simulink model "fsm_12B_with_contracts"  (R2019b)
settings: Solver=FixedStepDiscrete  StartTime=0.0  StopTime=10  RelTol=1e-3  EnableMultiTasking=on
model workspace (MAT data in the model file):
  ContractValidatorBlocksMap : containers.Map (value not decoded)
undefined symbols (not defined in the file): contractAfterSimulation, contractBeforeSimulation, ContractBlock, ContractGuaranteeBlock, ContractValidatorBlock, saveValidatorParameters
libraries: cocosimLibs x20
(part 1 of 2)
settings Model: Creator=elliocm  LastModifiedBy=hbourbou
settings DataIOCC: LimitDataPoints=on  SaveFormat=Array  ReturnWorkspaceOutputs=off
settings OptimizationCC: ExpressionDepthLimit=2147483647  LifeSpan=inf
settings DebuggingCC: UnderspecifiedInitializationDetection=Classic  MergeDetectMultiDrivingBlocksExec=none  SolverPrmCheckMsg=warning  StateNameClashWarn=warning  SFUnexpectedBacktrackingDiag=warning  SFNoUnconditionalDefaultTransitionDiag=warning  SFExecutionAtInitializationDiag=none  ArithmeticOperatorsInVariantConditions=warning
settings HardwareCC: ProdBitPerPointer=32  ProdBitPerSizeT=32  ProdBitPerPtrDiffT=32  ProdLargestAtomicFloat=None  ProdIntDivRoundTo=Undefined  ProdEndianess=Unspecified  ProdWordSize=32  ProdHWDeviceType=32-bit Generic
settings ModelReferenceCC: PropagateSignalLabelsOutOfModel=off
settings SFSimCC: SimUseLocalCustomCode=off  CustomCodeUndefinedFunction=UseInterfaceOnly
settings RTWCC: RTWUseLocalCustomCode=off
settings CodeAppCC: StateflowObjectComments=on
settings GRTTargetCC: TargetLangStandard=C89/C90 (ANSI)  GeneratePreprocessorConditionals=Disable all
settings ConfigComp: CovMetricSettings=dw  CovHtmlReporting=on  CovSaveCumulativeToWorkspaceVar=on  CovSaveSingleToWorkspaceVar=on  CovExternalEMLEnable=off

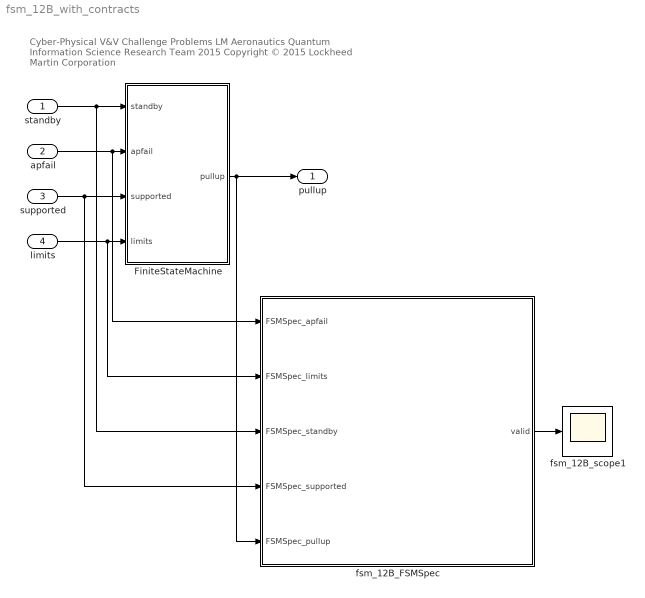
== system fsm_12B_with_contracts ==
  note: Cyber-Physical V&V Challenge Problems
      | LM Aeronautics Quantum Information Science Research Team 2015
      | Copyright © 2015 Lockheed Martin Corporation
  standby : Inport  OutDataTypeStr=boolean
  apfail : Inport  Port=2  OutDataTypeStr=boolean
  supported : Inport  Port=3  OutDataTypeStr=boolean
  limits : Inport  Port=4  OutDataTypeStr=boolean
  FiniteStateMachine : Subsystem
  fsm_12B_FSMSpec : Subsystem  mask(ContractBlock){ContractBlockType=ContractBlock}
      mask init:
      | set_param(gcb, 'LinkStatus', 'none');
      mask DialogControl DescTextVar Prompt: Contract block
      mask Display:
      | text(0.5, 0.5, '{\bf\fontsize{20}Contract}', 'hor', 'center', 'texmode','on');
      | blocks = find_system(gcb, 'LookUnderMasks','all', 'SearchDepth',1,'BlockType','Inport');
      | for i = 1 : length(blocks)
      |     blockName = get_param(blocks(i), 'Name');
      |     [path, blockName] = fileparts(char(blockName));
      |     port_label('input', i, blockName);
      | end
      | 
      | blocks = find_system(gcb, 'LookUnderMasks','all', 'SearchDepth',1,'BlockType','Outport');
      | for i = 1 : length(blocks)
      |     blockName = get_param(blocks(i), 'Name');
      |     [path, blockName] = fileparts(char(blockName));
      |     port_label('output', i, blockName);
      | end
  fsm_12B_scope1 : Scope
  pullup : Outport  VectorParamsAs1DForOutWhenUnconnected=off
  wires:
  standby/1 -> FiniteStateMachine/1(standby), fsm_12B_FSMSpec/3(FSMSpec_standby)
  apfail/1 -> FiniteStateMachine/2(apfail), fsm_12B_FSMSpec/1(FSMSpec_apfail)
  supported/1 -> FiniteStateMachine/3(supported), fsm_12B_FSMSpec/4(FSMSpec_supported)
  limits/1 -> FiniteStateMachine/4(limits), fsm_12B_FSMSpec/2(FSMSpec_limits)
  FiniteStateMachine/1(pullup) -> pullup/1, fsm_12B_FSMSpec/5(FSMSpec_pullup)
  fsm_12B_FSMSpec/1(valid) -> fsm_12B_scope1/1

== system fsm_12B_with_contracts/FiniteStateMachine ==
  note: 51
  standby : Inport
  apfail : Inport  Port=2
  supported : Inport  Port=3
  limits : Inport  Port=4
  FiniteStateMachine_FSM_AutopilotSpec1 : Subsystem  mask(ContractBlock){ContractBlockType=ContractBlock}
      mask init:
      | set_param(gcb, 'LinkStatus', 'none');
      mask DialogControl DescTextVar Prompt: Contract block
      mask Display:
      | text(0.5, 0.5, '{\bf\fontsize{20}Contract}', 'hor', 'center', 'texmode','on');
      | blocks = find_system(gcb, 'LookUnderMasks','all', 'SearchDepth',1,'BlockType','Inport');
      | for i = 1 : length(blocks)
      |     blockName = get_param(blocks(i), 'Name');
      |     [path, blockName] = fileparts(char(blockName));
      |     port_label('input', i, blockName);
      | end
      | 
      | blocks = find_system(gcb, 'LookUnderMasks','all', 'SearchDepth',1,'BlockType','Outport');
      | for i = 1 : length(blocks)
      |     blockName = get_param(blocks(i), 'Name');
      |     [path, blockName] = fileparts(char(blockName));
      |     port_label('output', i, blockName);
      | end
  FiniteStateMachine_FSM_SensorSpec : Subsystem  mask(ContractBlock){ContractBlockType=ContractBlock}
      mask init:
      | set_param(gcb, 'LinkStatus', 'none');
      mask DialogControl DescTextVar Prompt: Contract block
      mask Display:
      | text(0.5, 0.5, '{\bf\fontsize{20}Contract}', 'hor', 'center', 'texmode','on');
      | blocks = find_system(gcb, 'LookUnderMasks','all', 'SearchDepth',1,'BlockType','Inport');
      | for i = 1 : length(blocks)
      |     blockName = get_param(blocks(i), 'Name');
      |     [path, blockName] = fileparts(char(blockName));
      |     port_label('input', i, blockName);
      | end
      | 
      | blocks = find_system(gcb, 'LookUnderMasks','all', 'SearchDepth',1,'BlockType','Outport');
      | for i = 1 : length(blocks)
      |     blockName = get_param(blocks(i), 'Name');
      |     [path, blockName] = fileparts(char(blockName));
      |     port_label('output', i, blockName);
      | end
  Manager : Subsystem
  Sen : Subsystem
  Terminator : Terminator
  Terminator1 : Terminator
  Unit Delay : UnitDelay  SampleTime=-1  HasFrameUpgradeWarning=on
  Unit Delay1 : UnitDelay  SampleTime=-1  HasFrameUpgradeWarning=on
  Unit Delay2 : UnitDelay  InitialCondition=1  SampleTime=-1  HasFrameUpgradeWarning=on
  pullup : Outport  VectorParamsAs1DForOutWhenUnconnected=off
  wires:
  Manager/1(MODE) -> FiniteStateMachine_FSM_SensorSpec/1(FSM_SensorSpec_MODE), Sen/1(mode)
  Manager/4(STATE) -> FiniteStateMachine_FSM_AutopilotSpec1/6(FSM_AutopilotSpec_STATE), Unit Delay/1
  Unit Delay/1 -> FiniteStateMachine_FSM_AutopilotSpec1/4(FSM_AutopilotSpec_state), Manager/5(state)
  Manager/2(REQUEST) -> FiniteStateMachine_FSM_SensorSpec/3(FSM_SensorSpec_request), Sen/2(request)
  Unit Delay1/1 -> FiniteStateMachine_FSM_SensorSpec/4(FSM_SensorSpec_senstate), Sen/4(senstate)
  Unit Delay2/1 -> FiniteStateMachine_FSM_AutopilotSpec1/2(FSM_AutopilotSpec_good), Manager/4(good)
  Sen/2(SENSTATE) -> FiniteStateMachine_FSM_SensorSpec/5(FSM_SensorSpec_SENSTATE), Unit Delay1/1
  Sen/1(good) -> Unit Delay2/1
  Manager/3(PULL) -> pullup/1
  standby/1 -> FiniteStateMachine_FSM_AutopilotSpec1/3(FSM_AutopilotSpec_standby), Manager/1(standby)
  apfail/1 -> FiniteStateMachine_FSM_AutopilotSpec1/1(FSM_AutopilotSpec_apfail), Manager/2(apfail)
  supported/1 -> FiniteStateMachine_FSM_AutopilotSpec1/5(FSM_AutopilotSpec_supported), Manager/3(supported)
  limits/1 -> Sen/3(limits), FiniteStateMachine_FSM_SensorSpec/2(FSM_SensorSpec_limits)
  FiniteStateMachine_FSM_SensorSpec/1(valid) -> Terminator/1
  FiniteStateMachine_FSM_AutopilotSpec1/1(valid) -> Terminator1/1

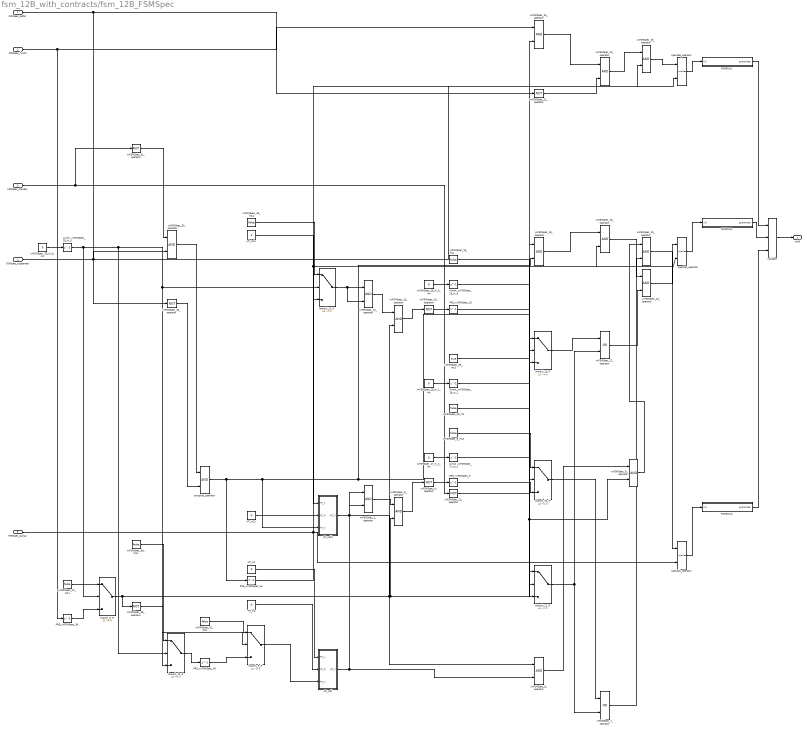
== system fsm_12B_with_contracts/fsm_12B_FSMSpec ==
  FSMSpec_apfail : Inport  OutDataTypeStr=boolean
  FSMSpec_limits : Inport  Port=2  OutDataTypeStr=boolean
  FSMSpec_standby : Inport  Port=3  OutDataTypeStr=boolean
  FSMSpec_supported : Inport  Port=4  OutDataTypeStr=boolean
  FSMSpec_pullup : Inport  Port=5  OutDataTypeStr=boolean
  Arrow_xxFSMSpec_26_ni_0 : Delay  DelayLength=1  InitialCondition=1
  Arrow_xxFSMSpec_27_ni_2 : Delay  DelayLength=1  InitialCondition=1
  Arrow_xxFSMSpec_28_ni_1 : Delay  DelayLength=1  InitialCondition=1
  Arrow_xxFSMSpec_33_ni_5 : Delay  DelayLength=1  InitialCondition=1
  FSM001v1 : Subsystem  mask(ContractGuaranteeBlock){ContractBlockType=ContractGuaranteeBlock}
      mask init:
      | set_param(gcb, 'LinkStatus', 'none');
      mask DialogControl DescTextVar Prompt: Guarantee block
  FSM001v2 : Subsystem  mask(ContractGuaranteeBlock){ContractBlockType=ContractGuaranteeBlock}
      mask init:
      | set_param(gcb, 'LinkStatus', 'none');
      mask DialogControl DescTextVar Prompt: Guarantee block
  FSM001v3 : Subsystem  mask(ContractGuaranteeBlock){ContractBlockType=ContractGuaranteeBlock}
      mask init:
      | set_param(gcb, 'LinkStatus', 'none');
      mask DialogControl DescTextVar Prompt: Guarantee block
  HT_In1 : Constant  Value=3  OutDataTypeStr=int32
  HT_In11 : Constant  Value=3  OutDataTypeStr=int32
  HT_In2 : Constant  Value=0  OutDataTypeStr=int32
  HT_In21 : Constant  Value=0  OutDataTypeStr=int32
  HT_call : Subsystem
  HT_call1 : Subsystem
  PRE_xxFSMSpec_{5,15,34,36,40} (5 alike) : Delay  DelayLength=1  InitialCondition=0
  autopilot_operator : Logic  AllPortsSameDT=off  OutDataTypeStr=boolean
  branch_10_IF : Switch  Criteria=u2 ~= 0
  branch_11_IF : Switch  Criteria=u2 ~= 0
  branch_12_IF : Switch  Criteria=u2 ~= 0
  branch_13_IF : Switch  Criteria=u2 ~= 0
  branch_14_IF : Switch  Criteria=u2 ~= 0
  branch_8_IF : Switch  Criteria=u2 ~= 0
  branch_9_IF : Switch  Criteria=u2 ~= 0
  spec166_operator : cocosimLibs/Implies  SystemSampleTime=-1  Latency=0  AutoFrameSizeCalculation=off
  spec194_operator : cocosimLibs/Implies  SystemSampleTime=-1  Latency=0  AutoFrameSizeCalculation=off
  spec222_operator : cocosimLibs/Implies  SystemSampleTime=-1  Latency=0  AutoFrameSizeCalculation=off
  validator : M-S-Function  LoadFcn=saveValidatorParameters(gcb);  InitFcn=contractBeforeSimulation();  StopFcn=contractAfterSimulation();  FunctionName=contract  mask(ContractValidatorBlock){assumePorts=0, guaranteePorts=3, modePorts=0, ContractBlockType=ContractValidatorBlock, createInportsCheckbox=off}
      mask prompts: assumePorts "Assume ports     :"; guaranteePorts "Guarantee ports :"; modePorts "Mode ports        :"; createInportsCheckbox "Create inports and connect them automatically"
      mask init:
      | set_param(gcb,'LinkStatus','none');
      | contract_callback('inputs_callback',gcb);
      mask DialogControl DescTextVar Prompt: The validator block implements the following logic: <br> <br> <b>Sofar</b>(assume<sub>1</sub> <b>&#8743;</b> assume<sub>2</sub> <b>&#8743;</b> ... assume<sub>k</sub>) <b>&rarr;</b> (guarantee<sub>1</sub> <b>&#8743;</b> guarantee<sub>2</sub> <b>&#8743;</b> ... guarantee<sub>m</sub> <b>&#8743;</b>  mode<sub>1</sub> <b>&#8743;</b> mode<sub>2</sub> <b>&#8743;</b> ... <b>&#8743;</b> mode<sub>n</sub> )<br> where mode<sub>i</sub> = require<sub>i</sub> <b>&rarr;</b> ensure<sub>i</sub>
      mask Display:
      | color('black');
      | port_label('input',1,'guarantee');
      | port_label('input',2,'guarantee');
      | port_label('input',3,'guarantee');
      | port_label('output',1,'valid');
  xxFSMSpec_10_operator : Logic  AllPortsSameDT=off  OutDataTypeStr=boolean
  xxFSMSpec_12_operator : Logic  AllPortsSameDT=off  OutDataTypeStr=boolean
  xxFSMSpec_13_operator : Logic  AllPortsSameDT=off  OutDataTypeStr=boolean
  xxFSMSpec_14_operator : Logic  Operator=NOT  AllPortsSameDT=off  OutDataTypeStr=boolean
  xxFSMSpec_16_rhs1 : Constant  Value=false  OutDataTypeStr=boolean
  xxFSMSpec_17_operator : Logic  Operator=OR  AllPortsSameDT=off  OutDataTypeStr=boolean
  xxFSMSpec_18_operator : Logic  AllPortsSameDT=off  OutDataTypeStr=boolean
  xxFSMSpec_19_operator : Logic  AllPortsSameDT=off  OutDataTypeStr=boolean
  xxFSMSpec_20_operator : Logic  AllPortsSameDT=off  OutDataTypeStr=boolean
  xxFSMSpec_21_operator : Logic  Operator=NOT  AllPortsSameDT=off  OutDataTypeStr=boolean
  xxFSMSpec_22_operator : Logic  Operator=NOT  AllPortsSameDT=off  OutDataTypeStr=boolean
  xxFSMSpec_23_operator : Logic  AllPortsSameDT=off  OutDataTypeStr=boolean
  xxFSMSpec_24_operator : Logic  AllPortsSameDT=off  OutDataTypeStr=boolean
  xxFSMSpec_25_operator : Logic  AllPortsSameDT=off  OutDataTypeStr=boolean
  xxFSMSpec_26_ni_0_init : Constant  Value=0  OutDataTypeStr=boolean
  xxFSMSpec_27_ni_2_init : Constant  Value=0  OutDataTypeStr=boolean
  xxFSMSpec_28_ni_1_init : Constant  Value=0  OutDataTypeStr=boolean
  xxFSMSpec_29_rhs : Constant  Value=false  OutDataTypeStr=boolean
  xxFSMSpec_29_rhs1 : Constant  Value=true  OutDataTypeStr=boolean
  xxFSMSpec_2_operator : Logic  AllPortsSameDT=off  OutDataTypeStr=boolean
  xxFSMSpec_30_operator : Logic  Operator=NOT  AllPortsSameDT=off  OutDataTypeStr=boolean
  xxFSMSpec_31_operator : Logic  Operator=NOT  AllPortsSameDT=off  OutDataTypeStr=boolean
  xxFSMSpec_32_operator : Logic  AllPortsSameDT=off  OutDataTypeStr=boolean
  xxFSMSpec_33_ni_5_init : Constant  Value=0  OutDataTypeStr=boolean
  xxFSMSpec_35_rhs1 : Constant  Value=false  OutDataTypeStr=boolean
  xxFSMSpec_37_rhs1 : Constant  Value=false  OutDataTypeStr=boolean
  xxFSMSpec_38_operator : Logic  Operator=NOT  AllPortsSameDT=off  OutDataTypeStr=boolean
  xxFSMSpec_39_rhs1 : Constant  Value=false  OutDataTypeStr=boolean
  xxFSMSpec_3_operator : Logic  AllPortsSameDT=off  OutDataTypeStr=boolean
  xxFSMSpec_41_rhs1 : Constant  Value=false  OutDataTypeStr=boolean
  xxFSMSpec_4_operator : Logic  Operator=NOT  AllPortsSameDT=off  OutDataTypeStr=boolean
  xxFSMSpec_6_rhs1 : Constant  Value=false  OutDataTypeStr=boolean
  xxFSMSpec_7_operator : Logic  Operator=OR  AllPortsSameDT=off  OutDataTypeStr=boolean
  xxFSMSpec_8_operator : Logic  AllPortsSameDT=off  OutDataTypeStr=boolean
  xxFSMSpec_9_operator : Logic  AllPortsSameDT=off  OutDataTypeStr=boolean
  valid : Outport
  wires:
  validator/1 -> valid/1
  xxFSMSpec_8_operator/1 -> xxFSMSpec_9_operator/1
  branch_10_IF/1 -> xxFSMSpec_7_operator/1
  xxFSMSpec_3_operator/1 -> xxFSMSpec_4_operator/1
  xxFSMSpec_2_operator/1 -> xxFSMSpec_3_operator/1
  xxFSMSpec_31_operator/1 -> xxFSMSpec_32_operator/1
  xxFSMSpec_24_operator/1 -> xxFSMSpec_25_operator/1
  xxFSMSpec_21_operator/1 -> xxFSMSpec_24_operator/2
  xxFSMSpec_23_operator/1 -> xxFSMSpec_24_operator/1
  xxFSMSpec_22_operator/1 -> xxFSMSpec_23_operator/2
  xxFSMSpec_17_operator/1 -> xxFSMSpec_20_operator/2
  xxFSMSpec_19_operator/1 -> xxFSMSpec_20_operator/1
  xxFSMSpec_18_operator/1 -> xxFSMSpec_19_operator/1
  branch_13_IF/1 -> xxFSMSpec_17_operator/1
  xxFSMSpec_13_operator/1 -> xxFSMSpec_14_operator/1
  xxFSMSpec_12_operator/1 -> xxFSMSpec_13_operator/1
  xxFSMSpec_7_operator/1 -> xxFSMSpec_10_operator/2
  xxFSMSpec_9_operator/1 -> xxFSMSpec_10_operator/1
  FSM001v3/1(guarantee) -> validator/3
  FSM001v2/1(guarantee) -> validator/2
  FSM001v1/1(guarantee) -> validator/1
  xxFSMSpec_10_operator/1 -> spec222_operator/1
  xxFSMSpec_20_operator/1 -> spec194_operator/1
  xxFSMSpec_25_operator/1 -> spec166_operator/1
  spec222_operator/1 -> FSM001v3/1(In1)
  spec194_operator/1 -> FSM001v2/1(In1)
  spec166_operator/1 -> FSM001v1/1(In1)
  PRE_xxFSMSpec_40/1 -> branch_9_IF/3
  xxFSMSpec_41_rhs1/1 -> branch_9_IF/1
  PRE_xxFSMSpec_36/1 -> branch_8_IF/3
  xxFSMSpec_37_rhs1/1 -> branch_8_IF/1
  xxFSMSpec_38_operator/1 -> branch_14_IF/3
  xxFSMSpec_39_rhs1/1 -> branch_14_IF/1
  PRE_xxFSMSpec_15/1 -> branch_13_IF/3
  Arrow_xxFSMSpec_26_ni_0/1 -> branch_13_IF/2
  xxFSMSpec_16_rhs1/1 -> branch_13_IF/1
  PRE_xxFSMSpec_34/1 -> branch_12_IF/3
  xxFSMSpec_35_rhs1/1 -> branch_12_IF/1
  xxFSMSpec_29_rhs/1 -> branch_11_IF/3
  Arrow_xxFSMSpec_28_ni_1/1 -> branch_11_IF/2
  xxFSMSpec_29_rhs1/1 -> branch_11_IF/1
  PRE_xxFSMSpec_5/1 -> branch_10_IF/3
  Arrow_xxFSMSpec_27_ni_2/1 -> branch_10_IF/2
  xxFSMSpec_6_rhs1/1 -> branch_10_IF/1
  xxFSMSpec_30_operator/1 -> autopilot_operator/2
  xxFSMSpec_32_operator/1 -> autopilot_operator/1
  xxFSMSpec_4_operator/1 -> PRE_xxFSMSpec_5/1
  branch_14_IF/1 -> PRE_xxFSMSpec_40/1
  xxFSMSpec_14_operator/1 -> PRE_xxFSMSpec_15/1
  HT_In21/1 -> HT_call1/2(HT_R)
  HT_In11/1 -> HT_call1/1(HT_L)
  branch_9_IF/1 -> HT_call/3(HT_X)
  HT_In2/1 -> HT_call/2(HT_R)
  HT_In1/1 -> HT_call/1(HT_L)
  xxFSMSpec_33_ni_5_init/1 -> Arrow_xxFSMSpec_33_ni_5/1
  xxFSMSpec_28_ni_1_init/1 -> Arrow_xxFSMSpec_28_ni_1/1
  xxFSMSpec_27_ni_2_init/1 -> Arrow_xxFSMSpec_27_ni_2/1
  xxFSMSpec_26_ni_0_init/1 -> Arrow_xxFSMSpec_26_ni_0/1
  branch_8_IF/1 -> xxFSMSpec_9_operator/2, xxFSMSpec_19_operator/2, xxFSMSpec_3_operator/2, xxFSMSpec_13_operator/2, xxFSMSpec_38_operator/1
  branch_12_IF/1 -> xxFSMSpec_18_operator/2, xxFSMSpec_12_operator/2
  HT_call/1(HT_Y) -> xxFSMSpec_8_operator/2, xxFSMSpec_2_operator/2
  HT_call1/1(HT_Y) -> xxFSMSpec_8_operator/1, xxFSMSpec_2_operator/1
  FSMSpec_pullup/1 -> spec194_operator/2, spec166_operator/2, spec222_operator/2
  FSMSpec_supported/1 -> xxFSMSpec_32_operator/2, xxFSMSpec_25_operator/2
  FSMSpec_apfail/1 -> xxFSMSpec_30_operator/1, xxFSMSpec_21_operator/1
  FSMSpec_limits/1 -> xxFSMSpec_23_operator/1, PRE_xxFSMSpec_36/1
  FSMSpec_standby/1 -> xxFSMSpec_31_operator/1, xxFSMSpec_22_operator/1
  branch_11_IF/1 -> xxFSMSpec_7_operator/2, xxFSMSpec_17_operator/2
  Arrow_xxFSMSpec_33_ni_5/1 -> branch_9_IF/2, branch_12_IF/2, branch_14_IF/2, branch_8_IF/2
  autopilot_operator/1 -> xxFSMSpec_18_operator/1, xxFSMSpec_12_operator/1, HT_call1/3(HT_X), PRE_xxFSMSpec_34/1

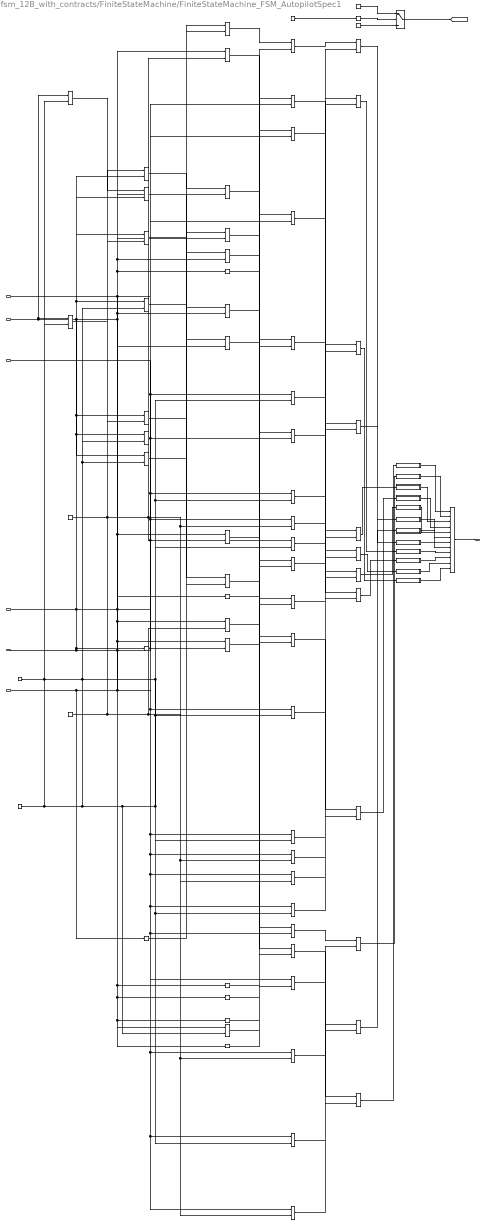
== system fsm_12B_with_contracts/FiniteStateMachine/FiniteStateMachine_FSM_AutopilotSpec1 ==
  FSM_AutopilotSpec_apfail : Inport  OutDataTypeStr=boolean
  FSM_AutopilotSpec_good : Inport  Port=2  OutDataTypeStr=boolean
  FSM_AutopilotSpec_standby : Inport  Port=3  OutDataTypeStr=boolean
  FSM_AutopilotSpec_state : Inport  Port=4  OutDataTypeStr=double
  FSM_AutopilotSpec_supported : Inport  Port=5  OutDataTypeStr=boolean
  FSM_AutopilotSpec_STATE : Inport  Port=6  OutDataTypeStr=double
  Arrow_xxFSM_AutopilotSpec_54_ni_7 : Delay  DelayLength=1  InitialCondition=1
  FSM002 : Subsystem  mask(ContractGuaranteeBlock){ContractBlockType=ContractGuaranteeBlock}
      mask init:
      | set_param(gcb, 'LinkStatus', 'none');
      mask DialogControl DescTextVar Prompt: Guarantee block
  FSM003 : Subsystem  mask(ContractGuaranteeBlock){ContractBlockType=ContractGuaranteeBlock}
      mask init:
      | set_param(gcb, 'LinkStatus', 'none');
      mask DialogControl DescTextVar Prompt: Guarantee block
  FSM003v2 : Subsystem  mask(ContractGuaranteeBlock){ContractBlockType=ContractGuaranteeBlock}
      mask init:
      | set_param(gcb, 'LinkStatus', 'none');
      mask DialogControl DescTextVar Prompt: Guarantee block
  FSM004 : Subsystem  mask(ContractGuaranteeBlock){ContractBlockType=ContractGuaranteeBlock}
      mask init:
      | set_param(gcb, 'LinkStatus', 'none');
      mask DialogControl DescTextVar Prompt: Guarantee block
  FSM004v2 : Subsystem  mask(ContractGuaranteeBlock){ContractBlockType=ContractGuaranteeBlock}
      mask init:
      | set_param(gcb, 'LinkStatus', 'none');
      mask DialogControl DescTextVar Prompt: Guarantee block
  FSM005 : Subsystem  mask(ContractGuaranteeBlock){ContractBlockType=ContractGuaranteeBlock}
      mask init:
      | set_param(gcb, 'LinkStatus', 'none');
      mask DialogControl DescTextVar Prompt: Guarantee block
  FSM006 : Subsystem  mask(ContractGuaranteeBlock){ContractBlockType=ContractGuaranteeBlock}
      mask init:
      | set_param(gcb, 'LinkStatus', 'none');
      mask DialogControl DescTextVar Prompt: Guarantee block
  FSM007 : Subsystem  mask(ContractGuaranteeBlock){ContractBlockType=ContractGuaranteeBlock}
      mask init:
      | set_param(gcb, 'LinkStatus', 'none');
      mask DialogControl DescTextVar Prompt: Guarantee block
  FSM007v2 : Subsystem  mask(ContractGuaranteeBlock){ContractBlockType=ContractGuaranteeBlock}
      mask init:
      | set_param(gcb, 'LinkStatus', 'none');
      mask DialogControl DescTextVar Prompt: Guarantee block
  FSM008v1 : Subsystem  mask(ContractGuaranteeBlock){ContractBlockType=ContractGuaranteeBlock}
      mask init:
      | set_param(gcb, 'LinkStatus', 'none');
      mask DialogControl DescTextVar Prompt: Guarantee block
  FSM008v2 : Subsystem  mask(ContractGuaranteeBlock){ContractBlockType=ContractGuaranteeBlock}
      mask init:
      | set_param(gcb, 'LinkStatus', 'none');
      mask DialogControl DescTextVar Prompt: Guarantee block
  FSM009 : Subsystem  mask(ContractGuaranteeBlock){ContractBlockType=ContractGuaranteeBlock}
      mask init:
      | set_param(gcb, 'LinkStatus', 'none');
      mask DialogControl DescTextVar Prompt: Guarantee block
  branch_6_IF : Switch  Criteria=u2 ~= 0
  spec129_operator : cocosimLibs/Implies  SystemSampleTime=-1  Latency=0  AutoFrameSizeCalculation=off
  spec143_operator : cocosimLibs/Implies  SystemSampleTime=-1  Latency=0  AutoFrameSizeCalculation=off
  spec160_operator : cocosimLibs/Implies  SystemSampleTime=-1  Latency=0  AutoFrameSizeCalculation=off
  spec182_operator : cocosimLibs/Implies  SystemSampleTime=-1  Latency=0  AutoFrameSizeCalculation=off
  spec198_operator : cocosimLibs/Implies  SystemSampleTime=-1  Latency=0  AutoFrameSizeCalculation=off
  spec212_operator : cocosimLibs/Implies  SystemSampleTime=-1  Latency=0  AutoFrameSizeCalculation=off
  spec233_operator : cocosimLibs/Implies  SystemSampleTime=-1  Latency=0  AutoFrameSizeCalculation=off
  spec254_operator : cocosimLibs/Implies  SystemSampleTime=-1  Latency=0  AutoFrameSizeCalculation=off
  spec271_operator : cocosimLibs/Implies  SystemSampleTime=-1  Latency=0  AutoFrameSizeCalculation=off
  spec287_operator : cocosimLibs/Implies  SystemSampleTime=-1  Latency=0  AutoFrameSizeCalculation=off
  spec309_operator : cocosimLibs/Implies  SystemSampleTime=-1  Latency=0  AutoFrameSizeCalculation=off
  spec326_operator : cocosimLibs/Implies  SystemSampleTime=-1  Latency=0  AutoFrameSizeCalculation=off
  validator : M-S-Function  LoadFcn=saveValidatorParameters(gcb);  InitFcn=contractBeforeSimulation();  StopFcn=contractAfterSimulation();  FunctionName=contract  mask(ContractValidatorBlock){assumePorts=0, guaranteePorts=12, modePorts=0, ContractBlockType=ContractValidatorBlock, createInportsCheckbox=off}
      mask prompts: assumePorts "Assume ports     :"; guaranteePorts "Guarantee ports :"; modePorts "Mode ports        :"; createInportsCheckbox "Create inports and connect them automatically"
      mask init:
      | set_param(gcb,'LinkStatus','none');
      | contract_callback('inputs_callback',gcb);
      mask DialogControl DescTextVar Prompt: The validator block implements the following logic: <br> <br> <b>Sofar</b>(assume<sub>1</sub> <b>&#8743;</b> assume<sub>2</sub> <b>&#8743;</b> ... assume<sub>k</sub>) <b>&rarr;</b> (guarantee<sub>1</sub> <b>&#8743;</b> guarantee<sub>2</sub> <b>&#8743;</b> ... guarantee<sub>m</sub> <b>&#8743;</b>  mode<sub>1</sub> <b>&#8743;</b> mode<sub>2</sub> <b>&#8743;</b> ... <b>&#8743;</b> mode<sub>n</sub> )<br> where mode<sub>i</sub> = require<sub>i</sub> <b>&rarr;</b> ensure<sub>i</sub>
      mask Display:
      | color('black');
      | port_label('input',1,'guarantee');
      | port_label('input',2,'guarantee');
      | port_label('input',3,'guarantee');
      | port_label('input',4,'guarantee');
      | port_label('input',5,'guarantee');
      | port_label('input',6,'guarantee');
      | port_label('input',7,'guarantee');
      | port_label('input',8,'guarantee');
      | port_label('input',9,'guarantee');
      | port_label('input',10,'guarantee');
      | port_label('input',11,'guarantee');
      | port_label('input',12,'guarantee');
      | port_label('output',1,'valid');
  xxFSM_AutopilotSpec_10_operator : Logic  AllPortsSameDT=off  OutDataTypeStr=boolean
  xxFSM_AutopilotSpec_11_operator : RelationalOperator  Operator===  OutDataTypeStr=boolean  RndMeth=Simplest
  xxFSM_AutopilotSpec_12_operator : RelationalOperator  Operator===  OutDataTypeStr=boolean  RndMeth=Simplest
  xxFSM_AutopilotSpec_13_operator : Logic  Operator=NOT  AllPortsSameDT=off  OutDataTypeStr=boolean
  xxFSM_AutopilotSpec_14_operator : Logic  AllPortsSameDT=off  OutDataTypeStr=boolean
  xxFSM_AutopilotSpec_15_operator : RelationalOperator  Operator===  OutDataTypeStr=boolean  RndMeth=Simplest
  xxFSM_AutopilotSpec_16_operator : RelationalOperator  Operator===  OutDataTypeStr=boolean  RndMeth=Simplest
  xxFSM_AutopilotSpec_17_operator : Logic  AllPortsSameDT=off  OutDataTypeStr=boolean
  xxFSM_AutopilotSpec_18_operator : Logic  AllPortsSameDT=off  OutDataTypeStr=boolean
  xxFSM_AutopilotSpec_19_operator : RelationalOperator  Operator===  OutDataTypeStr=boolean  RndMeth=Simplest
  xxFSM_AutopilotSpec_1_operator : RelationalOperator  Operator===  OutDataTypeStr=boolean  RndMeth=Simplest
  xxFSM_AutopilotSpec_20_operator : Logic  Operator=NOT  AllPortsSameDT=off  OutDataTypeStr=boolean
  xxFSM_AutopilotSpec_21_operator : Logic  Operator=NOT  AllPortsSameDT=off  OutDataTypeStr=boolean
  xxFSM_AutopilotSpec_22_operator : RelationalOperator  Operator===  OutDataTypeStr=boolean  RndMeth=Simplest
  xxFSM_AutopilotSpec_23_operator : Logic  AllPortsSameDT=off  OutDataTypeStr=boolean
  xxFSM_AutopilotSpec_24_operator : Logic  AllPortsSameDT=off  OutDataTypeStr=boolean
  xxFSM_AutopilotSpec_25_operator : RelationalOperator  Operator===  OutDataTypeStr=boolean  RndMeth=Simplest
  xxFSM_AutopilotSpec_26_operator : Logic  Operator=NOT  AllPortsSameDT=off  OutDataTypeStr=boolean
  xxFSM_AutopilotSpec_27_operator : Logic  Operator=NOT  AllPortsSameDT=off  OutDataTypeStr=boolean
  xxFSM_AutopilotSpec_28_operator : RelationalOperator  Operator===  OutDataTypeStr=boolean  RndMeth=Simplest
  xxFSM_AutopilotSpec_29_operator : Logic  AllPortsSameDT=off  OutDataTypeStr=boolean
  xxFSM_AutopilotSpec_2_operator : RelationalOperator  Operator===  OutDataTypeStr=boolean  RndMeth=Simplest
  xxFSM_AutopilotSpec_30_operator : Logic  AllPortsSameDT=off  OutDataTypeStr=boolean
  xxFSM_AutopilotSpec_31_operator : RelationalOperator  Operator===  OutDataTypeStr=boolean  RndMeth=Simplest
  xxFSM_AutopilotSpec_32_operator : RelationalOperator  Operator===  OutDataTypeStr=boolean  RndMeth=Simplest
  xxFSM_AutopilotSpec_33_operator : Logic  AllPortsSameDT=off  OutDataTypeStr=boolean
  xxFSM_AutopilotSpec_34_operator : RelationalOperator  Operator===  OutDataTypeStr=boolean  RndMeth=Simplest
  xxFSM_AutopilotSpec_35_operator : Logic  Operator=NOT  AllPortsSameDT=off  OutDataTypeStr=boolean
  xxFSM_AutopilotSpec_36_operator : RelationalOperator  Operator===  OutDataTypeStr=boolean  RndMeth=Simplest
  xxFSM_AutopilotSpec_37_operator : Logic  AllPortsSameDT=off  OutDataTypeStr=boolean
  xxFSM_AutopilotSpec_38_operator : RelationalOperator  Operator===  OutDataTypeStr=boolean  RndMeth=Simplest
  xxFSM_AutopilotSpec_39_operator : Logic  Operator=NOT  AllPortsSameDT=off  OutDataTypeStr=boolean
  xxFSM_AutopilotSpec_3_operator : Logic  AllPortsSameDT=off  OutDataTypeStr=boolean
  xxFSM_AutopilotSpec_40_operator : RelationalOperator  Operator===  OutDataTypeStr=boolean  RndMeth=Simplest
  xxFSM_AutopilotSpec_41_operator : Logic  AllPortsSameDT=off  OutDataTypeStr=boolean
  xxFSM_AutopilotSpec_42_operator : Logic  AllPortsSameDT=off  OutDataTypeStr=boolean
  xxFSM_AutopilotSpec_43_operator : Logic  AllPortsSameDT=off  OutDataTypeStr=boolean
  xxFSM_AutopilotSpec_44_operator : RelationalOperator  Operator===  OutDataTypeStr=boolean  RndMeth=Simplest
  xxFSM_AutopilotSpec_45_operator : RelationalOperator  Operator===  OutDataTypeStr=boolean  RndMeth=Simplest
  xxFSM_AutopilotSpec_46_operator : Logic  AllPortsSameDT=off  OutDataTypeStr=boolean
  xxFSM_AutopilotSpec_47_operator : Logic  AllPortsSameDT=off  OutDataTypeStr=boolean
  xxFSM_AutopilotSpec_48_operator : RelationalOperator  Operator===  OutDataTypeStr=boolean  RndMeth=Simplest
  xxFSM_AutopilotSpec_49_operator : RelationalOperator  Operator===  OutDataTypeStr=boolean  RndMeth=Simplest
  xxFSM_AutopilotSpec_4_operator : Logic  AllPortsSameDT=off  OutDataTypeStr=boolean
  xxFSM_AutopilotSpec_50_operator : Logic  AllPortsSameDT=off  OutDataTypeStr=boolean
  xxFSM_AutopilotSpec_51_operator : RelationalOperator  Operator===  OutDataTypeStr=boolean  RndMeth=Simplest
  xxFSM_AutopilotSpec_52_operator : RelationalOperator  Operator===  OutDataTypeStr=boolean  RndMeth=Simplest
  xxFSM_AutopilotSpec_53_operator : Logic  AllPortsSameDT=off  OutDataTypeStr=boolean
  xxFSM_AutopilotSpec_54_ni_7_init : Constant  Value=0  OutDataTypeStr=boolean
  xxFSM_AutopilotSpec_55_rhs : Constant  Value=false  OutDataTypeStr=boolean
  xxFSM_AutopilotSpec_55_rhs1 : Constant  Value=true  OutDataTypeStr=boolean
  xxFSM_AutopilotSpec_56_rhs : Constant  Value=2.0  OutDataTypeStr=double
  xxFSM_AutopilotSpec_57_rhs : Constant  Value=1.0  OutDataTypeStr=double
  xxFSM_AutopilotSpec_58_rhs : Constant  Value=3.0  OutDataTypeStr=double
  xxFSM_AutopilotSpec_59_rhs : Constant  Value=0.0  OutDataTypeStr=double
  xxFSM_AutopilotSpec_5_operator : RelationalOperator  Operator===  OutDataTypeStr=boolean  RndMeth=Simplest
  xxFSM_AutopilotSpec_6_operator : Logic  Operator=NOT  AllPortsSameDT=off  OutDataTypeStr=boolean
  xxFSM_AutopilotSpec_7_operator : RelationalOperator  Operator===  OutDataTypeStr=boolean  RndMeth=Simplest
  xxFSM_AutopilotSpec_8_operator : Logic  AllPortsSameDT=off  OutDataTypeStr=boolean
  xxFSM_AutopilotSpec_9_operator : Logic  AllPortsSameDT=off  OutDataTypeStr=boolean
  valid : Outport
  wires:
  validator/1 -> valid/1
  xxFSM_AutopilotSpec_8_operator/1 -> xxFSM_AutopilotSpec_9_operator/1
  xxFSM_AutopilotSpec_7_operator/1 -> xxFSM_AutopilotSpec_8_operator/1
  xxFSM_AutopilotSpec_52_operator/1 -> xxFSM_AutopilotSpec_53_operator/2
  xxFSM_AutopilotSpec_49_operator/1 -> xxFSM_AutopilotSpec_50_operator/1
  xxFSM_AutopilotSpec_3_operator/1 -> xxFSM_AutopilotSpec_4_operator/1
  xxFSM_AutopilotSpec_46_operator/1 -> xxFSM_AutopilotSpec_47_operator/1
  xxFSM_AutopilotSpec_45_operator/1 -> xxFSM_AutopilotSpec_46_operator/1
  xxFSM_AutopilotSpec_39_operator/1 -> xxFSM_AutopilotSpec_43_operator/2
  xxFSM_AutopilotSpec_42_operator/1 -> xxFSM_AutopilotSpec_43_operator/1
  xxFSM_AutopilotSpec_41_operator/1 -> xxFSM_AutopilotSpec_42_operator/1
  xxFSM_AutopilotSpec_40_operator/1 -> xxFSM_AutopilotSpec_41_operator/1
  xxFSM_AutopilotSpec_2_operator/1 -> xxFSM_AutopilotSpec_3_operator/1
  xxFSM_AutopilotSpec_35_operator/1 -> xxFSM_AutopilotSpec_37_operator/2
  xxFSM_AutopilotSpec_36_operator/1 -> xxFSM_AutopilotSpec_37_operator/1
  xxFSM_AutopilotSpec_32_operator/1 -> xxFSM_AutopilotSpec_33_operator/1
  xxFSM_AutopilotSpec_26_operator/1 -> xxFSM_AutopilotSpec_30_operator/2
  xxFSM_AutopilotSpec_29_operator/1 -> xxFSM_AutopilotSpec_30_operator/1
  xxFSM_AutopilotSpec_27_operator/1 -> xxFSM_AutopilotSpec_29_operator/2
  xxFSM_AutopilotSpec_28_operator/1 -> xxFSM_AutopilotSpec_29_operator/1
  xxFSM_AutopilotSpec_20_operator/1 -> xxFSM_AutopilotSpec_24_operator/2
  xxFSM_AutopilotSpec_23_operator/1 -> xxFSM_AutopilotSpec_24_operator/1
  xxFSM_AutopilotSpec_21_operator/1 -> xxFSM_AutopilotSpec_23_operator/2
  xxFSM_AutopilotSpec_22_operator/1 -> xxFSM_AutopilotSpec_23_operator/1
  xxFSM_AutopilotSpec_17_operator/1 -> xxFSM_AutopilotSpec_18_operator/1
  xxFSM_AutopilotSpec_16_operator/1 -> xxFSM_AutopilotSpec_17_operator/1
  xxFSM_AutopilotSpec_12_operator/1 -> xxFSM_AutopilotSpec_14_operator/2
  xxFSM_AutopilotSpec_13_operator/1 -> xxFSM_AutopilotSpec_14_operator/1
  xxFSM_AutopilotSpec_6_operator/1 -> xxFSM_AutopilotSpec_10_operator/2
  xxFSM_AutopilotSpec_9_operator/1 -> xxFSM_AutopilotSpec_10_operator/1
  FSM006/1(guarantee) -> validator/12
  FSM007v2/1(guarantee) -> validator/11
  FSM004/1(guarantee) -> validator/10
  FSM007/1(guarantee) -> validator/9
  FSM008v2/1(guarantee) -> validator/8
  FSM004v2/1(guarantee) -> validator/7
  FSM009/1(guarantee) -> validator/6
  FSM008v1/1(guarantee) -> validator/5
  FSM003v2/1(guarantee) -> validator/4
  FSM003/1(guarantee) -> validator/3
  FSM005/1(guarantee) -> validator/2
  FSM002/1(guarantee) -> validator/1
  xxFSM_AutopilotSpec_1_operator/1 -> spec326_operator/2
  xxFSM_AutopilotSpec_4_operator/1 -> spec326_operator/1
  xxFSM_AutopilotSpec_5_operator/1 -> spec309_operator/2
  xxFSM_AutopilotSpec_10_operator/1 -> spec309_operator/1
  xxFSM_AutopilotSpec_11_operator/1 -> spec287_operator/2
  xxFSM_AutopilotSpec_14_operator/1 -> spec287_operator/1
  xxFSM_AutopilotSpec_15_operator/1 -> spec271_operator/2
  xxFSM_AutopilotSpec_18_operator/1 -> spec271_operator/1
  xxFSM_AutopilotSpec_19_operator/1 -> spec254_operator/2
  xxFSM_AutopilotSpec_24_operator/1 -> spec254_operator/1
  xxFSM_AutopilotSpec_25_operator/1 -> spec233_operator/2
  xxFSM_AutopilotSpec_30_operator/1 -> spec233_operator/1
  xxFSM_AutopilotSpec_31_operator/1 -> spec212_operator/2
  xxFSM_AutopilotSpec_33_operator/1 -> spec212_operator/1
  xxFSM_AutopilotSpec_34_operator/1 -> spec198_operator/2
  xxFSM_AutopilotSpec_37_operator/1 -> spec198_operator/1
  xxFSM_AutopilotSpec_38_operator/1 -> spec182_operator/2
  xxFSM_AutopilotSpec_43_operator/1 -> spec182_operator/1
  xxFSM_AutopilotSpec_44_operator/1 -> spec160_operator/2
  xxFSM_AutopilotSpec_47_operator/1 -> spec160_operator/1
  xxFSM_AutopilotSpec_48_operator/1 -> spec143_operator/2
  xxFSM_AutopilotSpec_50_operator/1 -> spec143_operator/1
  xxFSM_AutopilotSpec_51_operator/1 -> spec129_operator/2
  xxFSM_AutopilotSpec_53_operator/1 -> spec129_operator/1
  spec326_operator/1 -> FSM006/1(In1)
  spec309_operator/1 -> FSM007v2/1(In1)
  spec287_operator/1 -> FSM004/1(In1)
  spec271_operator/1 -> FSM007/1(In1)
  spec254_operator/1 -> FSM008v2/1(In1)
  spec233_operator/1 -> FSM004v2/1(In1)
  spec212_operator/1 -> FSM009/1(In1)
  spec198_operator/1 -> FSM008v1/1(In1)
  spec182_operator/1 -> FSM003v2/1(In1)
  spec160_operator/1 -> FSM003/1(In1)
  spec143_operator/1 -> FSM005/1(In1)
  spec129_operator/1 -> FSM002/1(In1)
  xxFSM_AutopilotSpec_55_rhs/1 -> branch_6_IF/3
  Arrow_xxFSM_AutopilotSpec_54_ni_7/1 -> branch_6_IF/2
  xxFSM_AutopilotSpec_55_rhs1/1 -> branch_6_IF/1
  branch_6_IF/1 -> [FSM_AutopilotSpec_FTP]
  xxFSM_AutopilotSpec_54_ni_7_init/1 -> Arrow_xxFSM_AutopilotSpec_54_ni_7/1
  FSM_AutopilotSpec_apfail/1 -> xxFSM_AutopilotSpec_33_operator/2, xxFSM_AutopilotSpec_20_operator/1
  FSM_AutopilotSpec_standby/1 -> xxFSM_AutopilotSpec_6_operator/1, xxFSM_AutopilotSpec_26_operator/1, xxFSM_AutopilotSpec_35_operator/1, xxFSM_AutopilotSpec_39_operator/1, xxFSM_AutopilotSpec_53_operator/1, xxFSM_AutopilotSpec_50_operator/2, xxFSM_AutopilotSpec_3_operator/2, xxFSM_AutopilotSpec_21_operator/1
  xxFSM_AutopilotSpec_59_rhs/1 -> xxFSM_AutopilotSpec_19_operator/2, xxFSM_AutopilotSpec_15_operator/2, xxFSM_AutopilotSpec_5_operator/2, xxFSM_AutopilotSpec_34_operator/2, xxFSM_AutopilotSpec_52_operator/2, xxFSM_AutopilotSpec_45_operator/2, xxFSM_AutopilotSpec_40_operator/2
  FSM_AutopilotSpec_supported/1 -> xxFSM_AutopilotSpec_42_operator/2, xxFSM_AutopilotSpec_17_operator/2, xxFSM_AutopilotSpec_47_operator/2, xxFSM_AutopilotSpec_8_operator/2
  xxFSM_AutopilotSpec_56_rhs/1 -> xxFSM_AutopilotSpec_25_operator/2, xxFSM_AutopilotSpec_11_operator/2, xxFSM_AutopilotSpec_31_operator/2, xxFSM_AutopilotSpec_2_operator/2, xxFSM_AutopilotSpec_16_operator/2, xxFSM_AutopilotSpec_7_operator/2
  FSM_AutopilotSpec_STATE/1 -> xxFSM_AutopilotSpec_51_operator/1, xxFSM_AutopilotSpec_25_operator/1, xxFSM_AutopilotSpec_48_operator/1, xxFSM_AutopilotSpec_11_operator/1, xxFSM_AutopilotSpec_44_operator/1, xxFSM_AutopilotSpec_38_operator/1, xxFSM_AutopilotSpec_34_operator/1, xxFSM_AutopilotSpec_5_operator/1, xxFSM_AutopilotSpec_31_operator/1, xxFSM_AutopilotSpec_1_operator/1, xxFSM_AutopilotSpec_15_operator/1, xxFSM_AutopilotSpec_19_operator/1
  xxFSM_AutopilotSpec_57_rhs/1 -> xxFSM_AutopilotSpec_44_operator/2, xxFSM_AutopilotSpec_38_operator/2, xxFSM_AutopilotSpec_49_operator/2, xxFSM_AutopilotSpec_12_operator/2, xxFSM_AutopilotSpec_28_operator/2
  FSM_AutopilotSpec_state/1 -> xxFSM_AutopilotSpec_2_operator/1, xxFSM_AutopilotSpec_16_operator/1, xxFSM_AutopilotSpec_22_operator/1, xxFSM_AutopilotSpec_52_operator/1, xxFSM_AutopilotSpec_12_operator/1, xxFSM_AutopilotSpec_49_operator/1, xxFSM_AutopilotSpec_36_operator/1, xxFSM_AutopilotSpec_32_operator/1, xxFSM_AutopilotSpec_45_operator/1, xxFSM_AutopilotSpec_28_operator/1, xxFSM_AutopilotSpec_7_operator/1, xxFSM_AutopilotSpec_40_operator/1
  FSM_AutopilotSpec_good/1 -> xxFSM_AutopilotSpec_4_operator/2, xxFSM_AutopilotSpec_18_operator/2, xxFSM_AutopilotSpec_46_operator/2, xxFSM_AutopilotSpec_13_operator/1, xxFSM_AutopilotSpec_9_operator/2, xxFSM_AutopilotSpec_41_operator/2, xxFSM_AutopilotSpec_27_operator/1
  xxFSM_AutopilotSpec_58_rhs/1 -> xxFSM_AutopilotSpec_51_operator/2, xxFSM_AutopilotSpec_48_operator/2, xxFSM_AutopilotSpec_1_operator/2, xxFSM_AutopilotSpec_36_operator/2, xxFSM_AutopilotSpec_32_operator/2, xxFSM_AutopilotSpec_22_operator/2

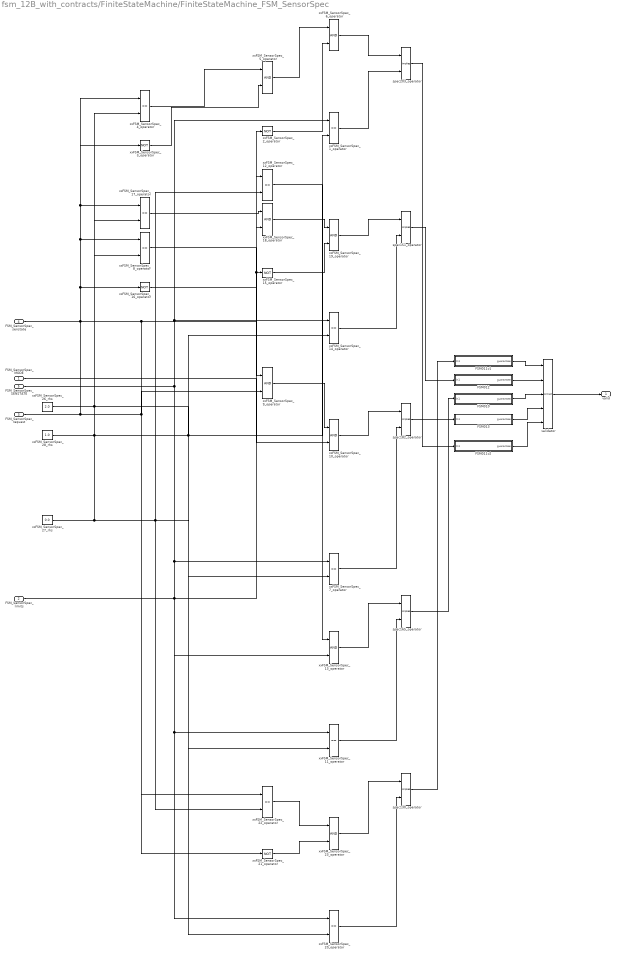
== system fsm_12B_with_contracts/FiniteStateMachine/FiniteStateMachine_FSM_SensorSpec ==
  FSM_SensorSpec_MODE : Inport  OutDataTypeStr=boolean
  FSM_SensorSpec_limits : Inport  Port=2  OutDataTypeStr=boolean
  FSM_SensorSpec_request : Inport  Port=3  OutDataTypeStr=boolean
  FSM_SensorSpec_senstate : Inport  Port=4  OutDataTypeStr=double
  FSM_SensorSpec_SENSTATE : Inport  Port=5  OutDataTypeStr=double
  FSM010 : Subsystem  mask(ContractGuaranteeBlock){ContractBlockType=ContractGuaranteeBlock}
      mask init:
      | set_param(gcb, 'LinkStatus', 'none');
      mask DialogControl DescTextVar Prompt: Guarantee block
  FSM011v1 : Subsystem  mask(ContractGuaranteeBlock){ContractBlockType=ContractGuaranteeBlock}
      mask init:
      | set_param(gcb, 'LinkStatus', 'none');
      mask DialogControl DescTextVar Prompt: Guarantee block
  FSM011v2 : Subsystem  mask(ContractGuaranteeBlock){ContractBlockType=ContractGuaranteeBlock}
      mask init:
      | set_param(gcb, 'LinkStatus', 'none');
      mask DialogControl DescTextVar Prompt: Guarantee block
  FSM012 : Subsystem  mask(ContractGuaranteeBlock){ContractBlockType=ContractGuaranteeBlock}
      mask init:
      | set_param(gcb, 'LinkStatus', 'none');
      mask DialogControl DescTextVar Prompt: Guarantee block
  FSM013 : Subsystem  mask(ContractGuaranteeBlock){ContractBlockType=ContractGuaranteeBlock}
      mask init:
      | set_param(gcb, 'LinkStatus', 'none');
      mask DialogControl DescTextVar Prompt: Guarantee block
  spec130_operator : cocosimLibs/Implies  SystemSampleTime=-1  Latency=0  AutoFrameSizeCalculation=off
  spec151_operator : cocosimLibs/Implies  SystemSampleTime=-1  Latency=0  AutoFrameSizeCalculation=off
  spec165_operator : cocosimLibs/Implies  SystemSampleTime=-1  Latency=0  AutoFrameSizeCalculation=off
  spec182_operator : cocosimLibs/Implies  SystemSampleTime=-1  Latency=0  AutoFrameSizeCalculation=off
  spec203_operator : cocosimLibs/Implies  SystemSampleTime=-1  Latency=0  AutoFrameSizeCalculation=off
  validator : M-S-Function  LoadFcn=saveValidatorParameters(gcb);  InitFcn=contractBeforeSimulation();  StopFcn=contractAfterSimulation();  FunctionName=contract  mask(ContractValidatorBlock){assumePorts=0, guaranteePorts=5, modePorts=0, ContractBlockType=ContractValidatorBlock, createInportsCheckbox=off}
      mask prompts: assumePorts "Assume ports     :"; guaranteePorts "Guarantee ports :"; modePorts "Mode ports        :"; createInportsCheckbox "Create inports and connect them automatically"
      mask init:
      | set_param(gcb,'LinkStatus','none');
      | contract_callback('inputs_callback',gcb);
      mask DialogControl DescTextVar Prompt: The validator block implements the following logic: <br> <br> <b>Sofar</b>(assume<sub>1</sub> <b>&#8743;</b> assume<sub>2</sub> <b>&#8743;</b> ... assume<sub>k</sub>) <b>&rarr;</b> (guarantee<sub>1</sub> <b>&#8743;</b> guarantee<sub>2</sub> <b>&#8743;</b> ... guarantee<sub>m</sub> <b>&#8743;</b>  mode<sub>1</sub> <b>&#8743;</b> mode<sub>2</sub> <b>&#8743;</b> ... <b>&#8743;</b> mode<sub>n</sub> )<br> where mode<sub>i</sub> = require<sub>i</sub> <b>&rarr;</b> ensure<sub>i</sub>
      mask Display:
      | color('black');
      | port_label('input',1,'guarantee');
      | port_label('input',2,'guarantee');
      | port_label('input',3,'guarantee');
      | port_label('input',4,'guarantee');
      | port_label('input',5,'guarantee');
      | port_label('output',1,'valid');
  xxFSM_SensorSpec_10_operator : Logic  AllPortsSameDT=off  OutDataTypeStr=boolean
  xxFSM_SensorSpec_11_operator : RelationalOperator  Operator===  OutDataTypeStr=boolean  RndMeth=Simplest
  xxFSM_SensorSpec_12_operator : RelationalOperator  Operator===  OutDataTypeStr=boolean  RndMeth=Simplest
  xxFSM_SensorSpec_13_operator : Logic  AllPortsSameDT=off  OutDataTypeStr=boolean
  xxFSM_SensorSpec_14_operator : RelationalOperator  Operator===  OutDataTypeStr=boolean  RndMeth=Simplest
  xxFSM_SensorSpec_15_operator : Logic  Operator=NOT  AllPortsSameDT=off  OutDataTypeStr=boolean
  xxFSM_SensorSpec_16_operator : Logic  Operator=NOT  AllPortsSameDT=off  OutDataTypeStr=boolean
  xxFSM_SensorSpec_17_operator : RelationalOperator  Operator===  OutDataTypeStr=boolean  RndMeth=Simplest
  xxFSM_SensorSpec_18_operator : Logic  AllPortsSameDT=off  OutDataTypeStr=boolean
  xxFSM_SensorSpec_19_operator : Logic  AllPortsSameDT=off  OutDataTypeStr=boolean
  xxFSM_SensorSpec_1_operator : RelationalOperator  Operator===  OutDataTypeStr=boolean  RndMeth=Simplest
  xxFSM_SensorSpec_20_operator : RelationalOperator  Operator===  OutDataTypeStr=boolean  RndMeth=Simplest
  xxFSM_SensorSpec_21_operator : Logic  Operator=NOT  AllPortsSameDT=off  OutDataTypeStr=boolean
  xxFSM_SensorSpec_22_operator : RelationalOperator  Operator===  OutDataTypeStr=boolean  RndMeth=Simplest
  xxFSM_SensorSpec_23_operator : Logic  AllPortsSameDT=off  OutDataTypeStr=boolean
  xxFSM_SensorSpec_26_rhs : Constant  Value=2.0  OutDataTypeStr=double
  xxFSM_SensorSpec_27_rhs : Constant  Value=0.0  OutDataTypeStr=double
  xxFSM_SensorSpec_28_rhs : Constant  Value=1.0  OutDataTypeStr=double
  xxFSM_SensorSpec_2_operator : Logic  Operator=NOT  AllPortsSameDT=off  OutDataTypeStr=boolean
  xxFSM_SensorSpec_3_operator : Logic  Operator=NOT  AllPortsSameDT=off  OutDataTypeStr=boolean
  xxFSM_SensorSpec_4_operator : RelationalOperator  Operator===  OutDataTypeStr=boolean  RndMeth=Simplest
  xxFSM_SensorSpec_5_operator : Logic  AllPortsSameDT=off  OutDataTypeStr=boolean
  xxFSM_SensorSpec_6_operator : Logic  AllPortsSameDT=off  OutDataTypeStr=boolean
  xxFSM_SensorSpec_7_operator : RelationalOperator  Operator===  OutDataTypeStr=boolean  RndMeth=Simplest
  xxFSM_SensorSpec_8_operator : RelationalOperator  Operator===  OutDataTypeStr=boolean  RndMeth=Simplest
  xxFSM_SensorSpec_9_operator : Logic  AllPortsSameDT=off  OutDataTypeStr=boolean
  valid : Outport
  wires:
  validator/1 -> valid/1
  xxFSM_SensorSpec_8_operator/1 -> xxFSM_SensorSpec_9_operator/1
  xxFSM_SensorSpec_2_operator/1 -> xxFSM_SensorSpec_6_operator/2
  xxFSM_SensorSpec_5_operator/1 -> xxFSM_SensorSpec_6_operator/1
  xxFSM_SensorSpec_3_operator/1 -> xxFSM_SensorSpec_5_operator/2
  xxFSM_SensorSpec_4_operator/1 -> xxFSM_SensorSpec_5_operator/1
  xxFSM_SensorSpec_21_operator/1 -> xxFSM_SensorSpec_23_operator/2
  xxFSM_SensorSpec_22_operator/1 -> xxFSM_SensorSpec_23_operator/1
  xxFSM_SensorSpec_15_operator/1 -> xxFSM_SensorSpec_19_operator/2
  xxFSM_SensorSpec_18_operator/1 -> xxFSM_SensorSpec_19_operator/1
  xxFSM_SensorSpec_16_operator/1 -> xxFSM_SensorSpec_18_operator/2
  xxFSM_SensorSpec_17_operator/1 -> xxFSM_SensorSpec_18_operator/1
  xxFSM_SensorSpec_12_operator/1 -> xxFSM_SensorSpec_13_operator/1
  FSM_SensorSpec_MODE/1 -> xxFSM_SensorSpec_10_operator/2
  xxFSM_SensorSpec_9_operator/1 -> xxFSM_SensorSpec_10_operator/1
  FSM011v2/1(guarantee) -> validator/5
  FSM013/1(guarantee) -> validator/4
  FSM010/1(guarantee) -> validator/3
  FSM012/1(guarantee) -> validator/2
  FSM011v1/1(guarantee) -> validator/1
  xxFSM_SensorSpec_1_operator/1 -> spec203_operator/2
  xxFSM_SensorSpec_6_operator/1 -> spec203_operator/1
  xxFSM_SensorSpec_7_operator/1 -> spec182_operator/2
  xxFSM_SensorSpec_10_operator/1 -> spec182_operator/1
  xxFSM_SensorSpec_11_operator/1 -> spec165_operator/2
  xxFSM_SensorSpec_13_operator/1 -> spec165_operator/1
  xxFSM_SensorSpec_14_operator/1 -> spec151_operator/2
  xxFSM_SensorSpec_19_operator/1 -> spec151_operator/1
  xxFSM_SensorSpec_20_operator/1 -> spec130_operator/2
  xxFSM_SensorSpec_23_operator/1 -> spec130_operator/1
  spec203_operator/1 -> FSM011v2/1(In1)
  spec182_operator/1 -> FSM013/1(In1)
  spec165_operator/1 -> FSM010/1(In1)
  spec151_operator/1 -> FSM012/1(In1)
  spec130_operator/1 -> FSM011v1/1(In1)
  xxFSM_SensorSpec_28_rhs/1 -> xxFSM_SensorSpec_20_operator/2, xxFSM_SensorSpec_1_operator/2, xxFSM_SensorSpec_14_operator/2, xxFSM_SensorSpec_8_operator/2
  FSM_SensorSpec_request/1 -> xxFSM_SensorSpec_9_operator/2, xxFSM_SensorSpec_21_operator/1, xxFSM_SensorSpec_3_operator/1, xxFSM_SensorSpec_16_operator/1
  xxFSM_SensorSpec_26_rhs/1 -> xxFSM_SensorSpec_17_operator/2, xxFSM_SensorSpec_11_operator/2
  FSM_SensorSpec_SENSTATE/1 -> xxFSM_SensorSpec_20_operator/1, xxFSM_SensorSpec_11_operator/1, xxFSM_SensorSpec_7_operator/1, xxFSM_SensorSpec_1_operator/1, xxFSM_SensorSpec_14_operator/1
  FSM_SensorSpec_limits/1 -> xxFSM_SensorSpec_2_operator/1, xxFSM_SensorSpec_15_operator/1, xxFSM_SensorSpec_13_operator/2
  xxFSM_SensorSpec_27_rhs/1 -> xxFSM_SensorSpec_7_operator/2, xxFSM_SensorSpec_22_operator/2, xxFSM_SensorSpec_12_operator/2, xxFSM_SensorSpec_4_operator/2
  FSM_SensorSpec_senstate/1 -> xxFSM_SensorSpec_22_operator/1, xxFSM_SensorSpec_12_operator/1, xxFSM_SensorSpec_4_operator/1, xxFSM_SensorSpec_17_operator/1, xxFSM_SensorSpec_8_operator/1

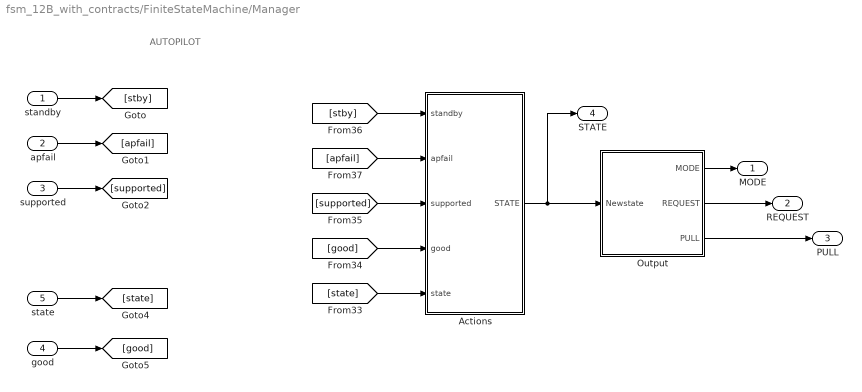
== system fsm_12B_with_contracts/FiniteStateMachine/Manager ==
  note: AUTOPILOT
  standby : Inport
  apfail : Inport  Port=2
  supported : Inport  Port=3
  good : Inport  Port=4
  state : Inport  Port=5
  Actions : Subsystem
  Output : Subsystem
  MODE : Outport  VectorParamsAs1DForOutWhenUnconnected=off
  REQUEST : Outport  Port=2  VectorParamsAs1DForOutWhenUnconnected=off
  PULL : Outport  Port=3  VectorParamsAs1DForOutWhenUnconnected=off
  STATE : Outport  Port=4  VectorParamsAs1DForOutWhenUnconnected=off
  wires:
  standby/1 -> [stby]
  supported/1 -> [supported]
  apfail/1 -> [apfail]
  state/1 -> [state]
  good/1 -> [good]
  Actions/1(STATE) -> STATE/1, Output/1(Newstate)
  [apfail] -> Actions/2(apfail)
  [state] -> Actions/5(state)
  [supported] -> Actions/3(supported)
  [good] -> Actions/4(good)
  [stby] -> Actions/1(standby)
  Output/1(MODE) -> MODE/1
  Output/2(REQUEST) -> REQUEST/1
  Output/3(PULL) -> PULL/1

== system fsm_12B_with_contracts/FiniteStateMachine/Sen ==
  note: SENSOR
  mode : Inport
  request : Inport  Port=2
  limits : Inport  Port=3
  senstate : Inport  Port=4
  Actions : Subsystem
  Output : Subsystem
  good : Outport  VectorParamsAs1DForOutWhenUnconnected=off
  SENSTATE : Outport  Port=2  VectorParamsAs1DForOutWhenUnconnected=off
  wires:
  request/1 -> [request]
  mode/1 -> [mode]
  limits/1 -> [limits]
  senstate/1 -> [senstate]
  Output/1(Good) -> good/1
  [request] -> Actions/2(request)
  [mode] -> Actions/1(mode)
  Actions/1(SENSTATE) -> Output/1(Newstate), SENSTATE/1
  [senstate] -> Actions/4(senstate)
  [limits] -> Actions/3(limits)

== system fsm_12B_with_contracts/fsm_12B_FSMSpec/FSM001v1 ==
  In1 : Inport
  guarantee : Outport  OutDataTypeStr=boolean
  wires:
  In1/1 -> guarantee/1

== system fsm_12B_with_contracts/fsm_12B_FSMSpec/FSM001v2 ==
  In1 : Inport
  guarantee : Outport  OutDataTypeStr=boolean
  wires:
  In1/1 -> guarantee/1

== system fsm_12B_with_contracts/fsm_12B_FSMSpec/FSM001v3 ==
  In1 : Inport
  guarantee : Outport  OutDataTypeStr=boolean
  wires:
  In1/1 -> guarantee/1

== system fsm_12B_with_contracts/fsm_12B_FSMSpec/HT_call ==
  HT_L : Inport
  HT_R : Inport  Port=2
  HT_X : Inport  Port=3  OutDataTypeStr=boolean
  OT_call : Subsystem
  Y_operator : Logic  Operator=NOT  AllPortsSameDT=off  OutDataTypeStr=boolean
  xxHT_1_operator : Logic  Operator=NOT  AllPortsSameDT=off  OutDataTypeStr=boolean
  HT_Y : Outport
  wires:
  Y_operator/1 -> HT_Y/1
  HT_X/1 -> xxHT_1_operator/1
  OT_call/1(OT_Y) -> Y_operator/1
  xxHT_1_operator/1 -> OT_call/3(OT_X)
  HT_R/1 -> OT_call/2(OT_R)
  HT_L/1 -> OT_call/1(OT_L)

== system fsm_12B_with_contracts/fsm_12B_FSMSpec/HT_call1 ==
  HT_L : Inport
  HT_R : Inport  Port=2
  HT_X : Inport  Port=3  OutDataTypeStr=boolean
  OT_call : Subsystem
  Y_operator : Logic  Operator=NOT  AllPortsSameDT=off  OutDataTypeStr=boolean
  xxHT_1_operator : Logic  Operator=NOT  AllPortsSameDT=off  OutDataTypeStr=boolean
  HT_Y : Outport
  wires:
  Y_operator/1 -> HT_Y/1
  HT_X/1 -> xxHT_1_operator/1
  OT_call/1(OT_Y) -> Y_operator/1
  xxHT_1_operator/1 -> OT_call/3(OT_X)
  HT_R/1 -> OT_call/2(OT_R)
  HT_L/1 -> OT_call/1(OT_L)

== system fsm_12B_with_contracts/FiniteStateMachine/FiniteStateMachine_FSM_AutopilotSpec1/FSM002 ==
  In1 : Inport
  guarantee : Outport  OutDataTypeStr=boolean
  wires:
  In1/1 -> guarantee/1

== system fsm_12B_with_contracts/FiniteStateMachine/FiniteStateMachine_FSM_AutopilotSpec1/FSM003 ==
  In1 : Inport
  guarantee : Outport  OutDataTypeStr=boolean
  wires:
  In1/1 -> guarantee/1

== system fsm_12B_with_contracts/FiniteStateMachine/FiniteStateMachine_FSM_AutopilotSpec1/FSM003v2 ==
  In1 : Inport
  guarantee : Outport  OutDataTypeStr=boolean
  wires:
  In1/1 -> guarantee/1

== system fsm_12B_with_contracts/FiniteStateMachine/FiniteStateMachine_FSM_AutopilotSpec1/FSM004 ==
  In1 : Inport
  guarantee : Outport  OutDataTypeStr=boolean
  wires:
  In1/1 -> guarantee/1

== system fsm_12B_with_contracts/FiniteStateMachine/FiniteStateMachine_FSM_AutopilotSpec1/FSM004v2 ==
  In1 : Inport
  guarantee : Outport  OutDataTypeStr=boolean
  wires:
  In1/1 -> guarantee/1

== system fsm_12B_with_contracts/FiniteStateMachine/FiniteStateMachine_FSM_AutopilotSpec1/FSM005 ==
  In1 : Inport
  guarantee : Outport  OutDataTypeStr=boolean
  wires:
  In1/1 -> guarantee/1
